simulink model "feature2_cc"  (R2020b)
settings: Solver=VariableStepAuto  StartTime=0.0  StopTime=inf  RelTol=1e-3
settings Model: Creator=99003757  LastModifiedBy=99003757

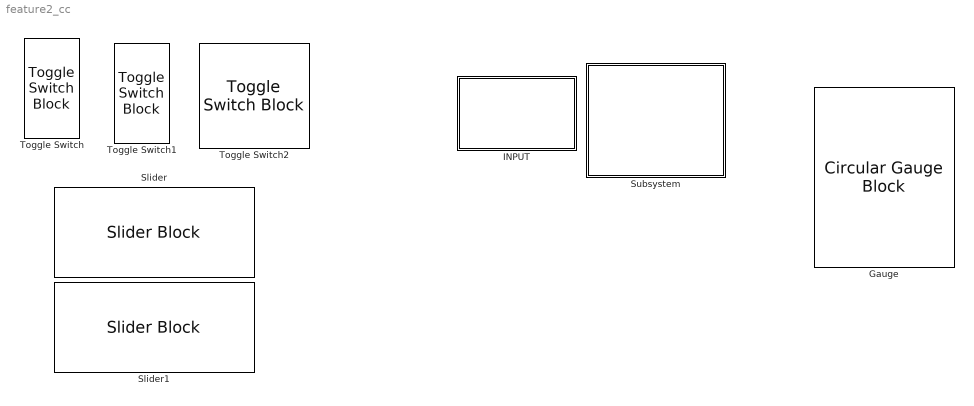
== system feature2_cc ==
  Gauge : CircularGaugeBlock
  INPUT : Subsystem
  Slider : SliderBlock
  Slider1 : SliderBlock
  Subsystem : Subsystem
  Toggle Switch : ToggleSwitchBlock
      settings: Values={{'Off', 'On'}, [0 1]}
  Toggle Switch1 : ToggleSwitchBlock
      settings: Values={{'Off', 'On'}, [0 1]}
  Toggle Switch2 : ToggleSwitchBlock
      settings: Values={{'Off', 'On'}, [0 1]}

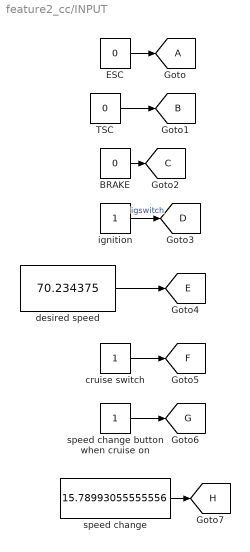
== system feature2_cc/INPUT ==
  BRAKE : Constant  Value=0
  ESC : Constant  Value=0
  TSC : Constant  Value=0
  cruise switch : Constant
  desired speed : Constant  Value=70.234375
  "ignition " : Constant
  speed change : Constant  Value=15.78993055555556
  "speed change button when cruise on " : Constant
  tag scope: A=global, B=global, C=global, D=global, E=global, F=global, G=global, H=global
  wires:
  "ignition "/1 -> [D]  "igswitch"
  cruise switch/1 -> [F]
  BRAKE/1 -> [C]
  desired speed/1 -> [E]
  "speed change button when cruise on "/1 -> [G]
  TSC/1 -> [B]
  ESC/1 -> [A]
  speed change/1 -> [H]

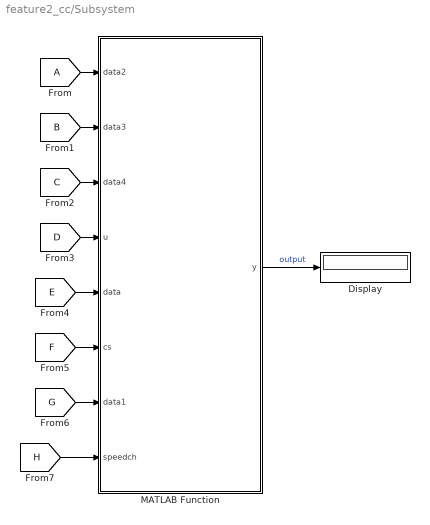
== system feature2_cc/Subsystem ==
  Display : Display
  MATLAB Function : MATLAB Function  TreatAsAtomicUnit=on
  wires:
  MATLAB Function/1(y) -> Display/1  "output"
  [H] -> MATLAB Function/8(speedch)
  [A] -> MATLAB Function/1(data2)
  [F] -> MATLAB Function/6(cs)
  [C] -> MATLAB Function/3(data4)
  [E] -> MATLAB Function/5(data)
  [G] -> MATLAB Function/7(data1)
  [B] -> MATLAB Function/2(data3)
  [D] -> MATLAB Function/4(u)

== matlab function feature2_cc/Subsystem/MATLAB Function ==
  data: data2 input; data3 input; data4 input; u input; y output; data input; cs input; data1 input; speedch input
function y = fcn(data2, data3, data4, u, data, cs, data1, speedch)

if (u==1&& data2==0 &&data3==0 && data4==0)
    if (cs ==1 && data>40 && data1==1)
        y= data+speedch;
    else
        y=data;
    end
      
else
    y=0;
end
